simulink model "WiperControlLogic"  (R2022b)
settings: Solver=FixedStepDiscrete  StartTime=0.0  StopTime=10.0  FixedStep=0.1  RelTol=1e-3
settings Model: Creator=Abdelrhman Shaban  LastModifiedBy=Abdelrhman Shaban

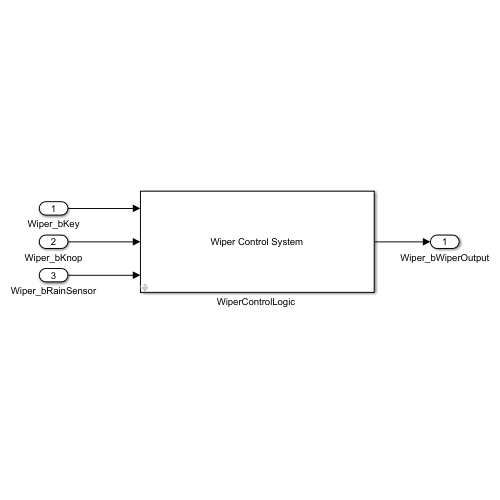
[thumbnail: Simulink's stored preview of the top-level diagram]
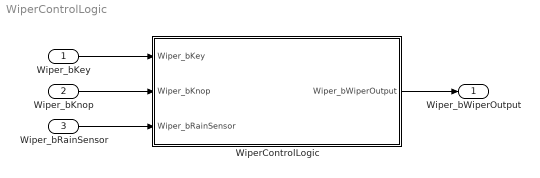
== system WiperControlLogic ==
  Wiper_bKey : Inport  OutDataTypeStr=boolean
  Wiper_bKnop : Inport  Port=2  OutDataTypeStr=boolean
  Wiper_bRainSensor : Inport  Port=3  OutDataTypeStr=boolean
  "WiperControlLogic " : Subsystem
      mask Display: disp('Wiper Control System');
  Wiper_bWiperOutput : Outport  OutDataTypeStr=boolean
  wires:
  "WiperControlLogic "/1(Wiper_bWiperOutput) -> Wiper_bWiperOutput/1
  Wiper_bRainSensor/1 -> "WiperControlLogic "/3(Wiper_bRainSensor)
  Wiper_bKnop/1 -> "WiperControlLogic "/2(Wiper_bKnop)
  Wiper_bKey/1 -> "WiperControlLogic "/1(Wiper_bKey)

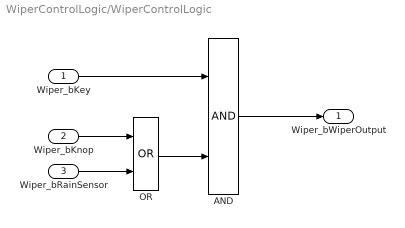
== system WiperControlLogic/WiperControlLogic  ==
  Wiper_bKey : Inport  OutDataTypeStr=boolean
  Wiper_bKnop : Inport  Port=2  OutDataTypeStr=boolean
  Wiper_bRainSensor : Inport  Port=3  OutDataTypeStr=boolean
  AND : Logic  AllPortsSameDT=off  OutDataTypeStr=boolean
  OR : Logic  Operator=OR  AllPortsSameDT=off  OutDataTypeStr=boolean
  Wiper_bWiperOutput : Outport  OutDataTypeStr=boolean
  wires:
  Wiper_bKnop/1 -> OR/1
  Wiper_bRainSensor/1 -> OR/2
  OR/1 -> AND/2
  Wiper_bKey/1 -> AND/1
  AND/1 -> Wiper_bWiperOutput/1
